simulink model "autosar_bsw_override_test"  (R2022b)
settings: Solver=VariableStepAuto  StartTime=0.0  StopTime=8  RelTol=1e-3
libraries: autosarlibdem x5, simulink x4
settings Model: Creator=The MathWorks, Inc.  LastModifiedBy=The MathWorks, Inc.
settings SolverCC: MaxZcPerStep=1
settings OptimizationCC: DefaultParameterBehavior=Inlined  EnhancedBackFolding=on  PassReuseOutputArgsAs=Individual arguments  ZeroExternalMemoryAtStartup=off  ZeroInternalMemoryAtStartup=off  OptimizeBlockOrder=speed  DifferentSizesBufferReuse=on  OptimizationCustomize=off  EfficientTunableParamExpr=on
settings DebuggingCC: ParameterTunabilityLossMsg=error
settings ModelReferenceCC: EnableRefExpFcnMdlSchedulingChecks=on
settings SFSimCC: MATLABDynamicMemAlloc=off
settings RTWCC: Description=AUTOSAR  SystemTargetFile=autosar.tlc  GenCodeOnly=on  TemplateMakefile=ert_default_tmf  DLArmComputeVersion=19.05
settings CodeAppCC: ForceParamTrailComments=on  IgnoreCustomStorageClasses=off  OperatorAnnotations=on  SimulinkDataObjDesc=on  SFDataObjDesc=on  InsertBlockDesc=on
settings STFCustomTargetCC: TargetLangStandard=C99 (ISO)  MultiwordLength=256  ParMdlRefBuildCompliant=on  CompOptLevelCompliant=on  IncludeMdlTerminateFcn=off  CombineOutputUpdateFcns=on  SuppressErrorStatus=on  ERTCustomFileBanners=on  SupportNonFinite=off  SupportComplex=off  SupportContinuousTime=off  SupportNonInlinedSFcns=off  RemoveResetFunc=on  MATLABClassNameForMDSCustomization=Simulink.SoftwareTarget.ERTCustomization  AutosarCompliant=on  UseToolchainInfoCompliant=on  LookupTableObjectStructAxisOrder=2,1,3,4,...  LUTObjectStructOrderEvenSpacing=Size,Table,Breakpoints  SystemTargetFile=autosar.tlc
settings ERTTargetCC: TargetLangStandard=C99 (ISO)  ConcurrentExecutionCompliant=off  IncludeMdlTerminateFcn=off  SuppressErrorStatus=on  SupportNonFinite=off  SupportComplex=off  ModelStepFunctionPrototypeControlCompliant=off  CPPClassGenCompliant=off  AutosarCompliant=on  LookupTableObjectStructAxisOrder=2,1,3,4,...  LUTObjectStructOrderEvenSpacing=Size,Table,Breakpoints  InlinedParameterPlacement=NonHierarchical  ERTCustomFileTemplate=example_file_process.tlc
settings ConfigComp: CovEnableCumulative=off

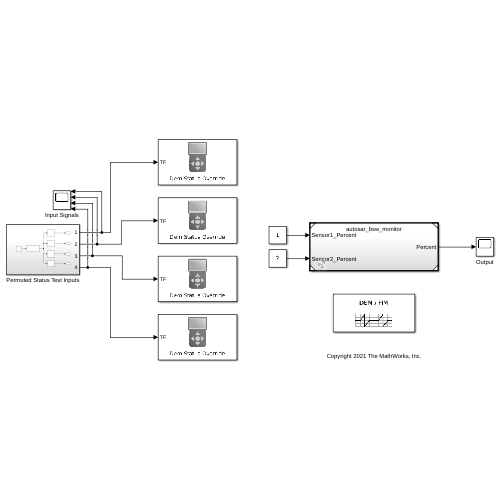
[thumbnail: Simulink's stored preview of the top-level diagram]
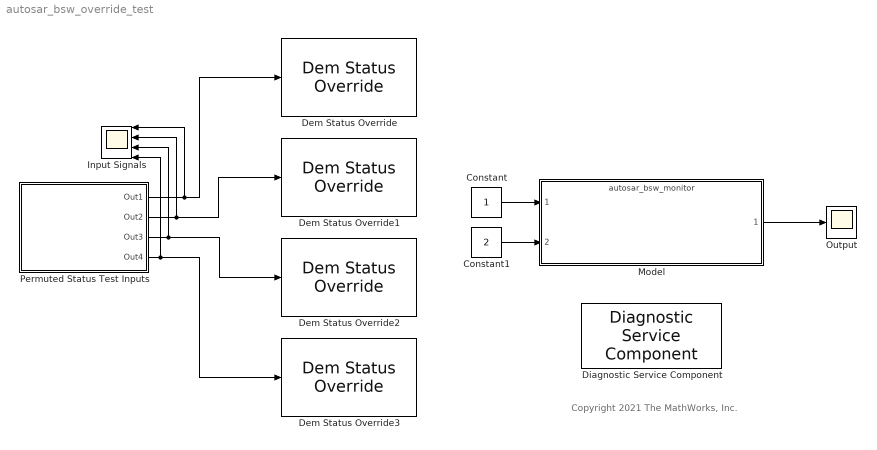
== system autosar_bsw_override_test ==
  note: Copyright 2021 The MathWorks, Inc.
  Constant : Constant  OutDataTypeStr=single
  Constant1 : Constant  Value=2  OutDataTypeStr=single
  Dem Status Override : autosarlibdem/Dem Status Override  Priority=1  EventId=1  TF_Source=Input port  TF_Value=off  TFTOC_Source=Dialog  TFTOC_Value=off  PDTC_Source=Dialog  PDTC_Value=off  CDTC_Source=Dialog  CDTC_Value=off  TNCSLC_Source=Dialog  TNCSLC_Value=off  TFSLC_Source=Dialog  TFSLC_Value=off  TNCTOC_Source=Dialog  TNCTOC_Value=off  WIR_Source=Dialog  WIR_Value=off
  Dem Status Override1 : autosarlibdem/Dem Status Override  Priority=1  EventId=2  TF_Source=Input port  TF_Value=off  TFTOC_Source=Dialog  TFTOC_Value=off  PDTC_Source=Dialog  PDTC_Value=off  CDTC_Source=Dialog  CDTC_Value=off  TNCSLC_Source=Dialog  TNCSLC_Value=off  TFSLC_Source=Dialog  TFSLC_Value=off  TNCTOC_Source=Dialog  TNCTOC_Value=off  WIR_Source=Dialog  WIR_Value=off
  Dem Status Override2 : autosarlibdem/Dem Status Override  Priority=1  EventId=3  TF_Source=Input port  TF_Value=off  TFTOC_Source=Dialog  TFTOC_Value=off  PDTC_Source=Dialog  PDTC_Value=off  CDTC_Source=Dialog  CDTC_Value=off  TNCSLC_Source=Dialog  TNCSLC_Value=off  TFSLC_Source=Dialog  TFSLC_Value=off  TNCTOC_Source=Dialog  TNCTOC_Value=off  WIR_Source=Dialog  WIR_Value=off
  Dem Status Override3 : autosarlibdem/Dem Status Override  Priority=1  EventId=4  TF_Source=Input port  TF_Value=off  TFTOC_Source=Dialog  TFTOC_Value=off  PDTC_Source=Dialog  PDTC_Value=off  CDTC_Source=Dialog  CDTC_Value=off  TNCSLC_Source=Dialog  TNCSLC_Value=off  TFSLC_Source=Dialog  TFSLC_Value=off  TNCTOC_Source=Dialog  TNCTOC_Value=off  WIR_Source=Dialog  WIR_Value=off
  Diagnostic Service Component : autosarlibdem/Diagnostic Service Component  ClientPortNames={'TPS', 'TPS1StuckHigh', 'TPS1StuckLow', 'TPS2StuckHigh', 'TPS2StuckLow'}  ClientPortPortDefinedArguments={'5', '1', '2', '3', '4'}  MaxEventId=5  MaxFID=1  DemDebounceCounterIncrementStepSize=1  DemDebounceCounterDecrementStepSize=1  DemDebounceCounterFailedThreshold=2  DemDebounceCounterPassedThreshold=-1  InhibitionMatrix=[0 0 0 0 0 0 0 0 0 0 0;0 0 0 0 0 0 0 0 0 0 0;0 0 0 0 0 0 0 0 0 0 0;0 0 0 0 0 0 0 0 0 0 0;0 0 0 0 0 0 0 0 0 0 0;0 0 0 0 0 0 0 0 0 0 0;0 0 0 0 0 0 0 0 0 0 0;0 0 0 0 0 0 0 0 0 0 0;0 0 0 0 0 0 0 0 0 0 0;0 0 0 0 0 0 0 0 0 0 0;0 0 0 0 0 0 0 0 0 0 0]  EnableConditionIndexes=zeros(257,'uint8')  StorageConditionIndexes=zeros(257,'uint8')
  Input Signals : Scope  NumInputPorts=4
  Model : ModelReference  ModelNameDialog=autosar_bsw_monitor  SimulationMode=Normal  ModelReferenceVersion=7.0
  Output : Scope
  Permuted Status Test Inputs : Subsystem
  wires:
  Constant/1 -> Model/1
  Constant1/1 -> Model/2
  Model/1 -> Output/1
  Permuted Status Test Inputs/1(Out1) -> Dem Status Override/1, Input Signals/1
  Permuted Status Test Inputs/2(Out2) -> Dem Status Override1/1, Input Signals/2
  Permuted Status Test Inputs/4(Out4) -> Dem Status Override3/1, Input Signals/4
  Permuted Status Test Inputs/3(Out3) -> Dem Status Override2/1, Input Signals/3

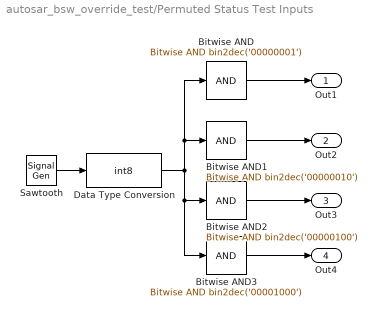
== system autosar_bsw_override_test/Permuted Status Test Inputs ==
  Bitwise AND : simulink/Logic and Bit Operations/Bitwise Operator  logicop=AND  UseBitMask=on  BitMask=bin2dec('00000001')  BitMaskRealWorld=Stored Integer
  Bitwise AND1 : simulink/Logic and Bit Operations/Bitwise Operator  logicop=AND  UseBitMask=on  BitMask=bin2dec('00000010')  BitMaskRealWorld=Stored Integer
  Bitwise AND2 : simulink/Logic and Bit Operations/Bitwise Operator  logicop=AND  UseBitMask=on  BitMask=bin2dec('00000100')  BitMaskRealWorld=Stored Integer
  Bitwise AND3 : simulink/Logic and Bit Operations/Bitwise Operator  logicop=AND  UseBitMask=on  BitMask=bin2dec('00001000')  BitMaskRealWorld=Stored Integer
  Data Type Conversion : DataTypeConversion  OutDataTypeStr=int8  SaturateOnIntegerOverflow=off  RndMeth=Floor
  Sawtooth : SignalGenerator  WaveForm=sawtooth  Amplitude=8  Frequency=0.125
  Out1 : Outport
  Out2 : Outport  Port=2
  Out3 : Outport  Port=3
  Out4 : Outport  Port=4
  wires:
  Bitwise AND3/1 -> Out4/1
  Sawtooth/1 -> Data Type Conversion/1
  Data Type Conversion/1 -> Bitwise AND/1, Bitwise AND1/1, Bitwise AND3/1, Bitwise AND2/1
  Bitwise AND2/1 -> Out3/1
  Bitwise AND/1 -> Out1/1
  Bitwise AND1/1 -> Out2/1
